simulink model "fec_ber_hw"  (R2020b)
settings: Solver=FixedStepDiscrete  StartTime=0.0  StopTime=T/2  RelTol=1e-3
values from neighbouring files (symbols this model uses):
  aximm_awgn_reset = 0    [setup.m]
  aximm_bit_count_reset = 0    [setup.m]
  aximm_bits = n_blocks * k    (= 3200)    [setup.m]
  aximm_ctrl_word_dec = 0    [setup.m]
  aximm_ctrl_word_enc = 0    [setup.m]
  aximm_enable = 1    [setup.m]
  aximm_length = k * n_blocks    (= 3200)    [setup.m]
  aximm_length_dec = n    (= 160)    [setup.m]
  aximm_length_enc = k    (= 80)    [setup.m]
  aximm_llr_mag_reset = 0    [setup.m]
  aximm_llr_scale = (1/noise_var) * llr_scale    (= 1000)    [setup.m]
  aximm_load_dec = 1    [setup.m]
  aximm_load_enc = 1    [setup.m]
  aximm_noise_std = sqrt(noise_var)    [setup.m]
  aximm_reset = 0    [setup.m]
  d = sqrt(-2*log([0:1/4095:1]))    [setup.m]
  fs = 160e6    (= 160000000)    [setup.m]
  llr_scale = 7.75/7.75    (= 1)    [setup.m]
libraries: simulink x450, hdlsllib x190, commseqgen3 x20, dspsigops x17, lib_rfsoc_fec x5, commblkcod2 x3
(part 20 of 22)

== system fec_ber_hw/Soft Demodulation/SSR Soft Demodulation Lane 1/Soft Demodulation 10/Subsystem2/get_min2 ==
  a : Inport
  b : Inport  Port=2
  Compare To Zero : simulink/Logic and Bit Operations/Compare To Zero  relop=<=  OutDataTypeStr=boolean
  Multiport Switch2 : MultiPortSwitch  DataPortOrder=Zero-based contiguous  Inputs=2  zeroidx=on
  Subtract18 : Sum  Inputs=+-  OutDataTypeStr=fixdt(1,(w+1)*2+2,f*2)  SaturateOnIntegerOverflow=on
  min : Outport
  wires:
  Compare To Zero/1 -> Multiport Switch2/1
  Multiport Switch2/1 -> min/1
  a/1 -> Subtract18/1, Multiport Switch2/3
  b/1 -> Multiport Switch2/2, Subtract18/2
  Subtract18/1 -> Compare To Zero/1

== system fec_ber_hw/Soft Demodulation/SSR Soft Demodulation Lane 1/Soft Demodulation 10/Subsystem2/get_min3 ==
  a : Inport
  b : Inport  Port=2
  Compare To Zero : simulink/Logic and Bit Operations/Compare To Zero  relop=<=  OutDataTypeStr=boolean
  Multiport Switch2 : MultiPortSwitch  DataPortOrder=Zero-based contiguous  Inputs=2  zeroidx=on
  Subtract18 : Sum  Inputs=+-  OutDataTypeStr=fixdt(1,(w+1)*2+2,f*2)  SaturateOnIntegerOverflow=on
  min : Outport
  wires:
  Subtract18/1 -> Compare To Zero/1
  b/1 -> Subtract18/2, Multiport Switch2/2
  a/1 -> Multiport Switch2/3, Subtract18/1
  Multiport Switch2/1 -> min/1
  Compare To Zero/1 -> Multiport Switch2/1

== system fec_ber_hw/Soft Demodulation/SSR Soft Demodulation Lane 1/Soft Demodulation 10/Subsystem2/get_min4 ==
  a : Inport
  b : Inport  Port=2
  Compare To Zero : simulink/Logic and Bit Operations/Compare To Zero  relop=<=  OutDataTypeStr=boolean
  Multiport Switch2 : MultiPortSwitch  DataPortOrder=Zero-based contiguous  Inputs=2  zeroidx=on
  Subtract18 : Sum  Inputs=+-  OutDataTypeStr=fixdt(1,(w+1)*2+2,f*2)  SaturateOnIntegerOverflow=on
  min : Outport
  wires:
  Compare To Zero/1 -> Multiport Switch2/1
  Multiport Switch2/1 -> min/1
  a/1 -> Subtract18/1, Multiport Switch2/3
  b/1 -> Multiport Switch2/2, Subtract18/2
  Subtract18/1 -> Compare To Zero/1

== system fec_ber_hw/Soft Demodulation/SSR Soft Demodulation Lane 1/Soft Demodulation 10/Subsystem2/get_min5 ==
  a : Inport
  b : Inport  Port=2
  Compare To Zero : simulink/Logic and Bit Operations/Compare To Zero  relop=<=  OutDataTypeStr=boolean
  Multiport Switch2 : MultiPortSwitch  DataPortOrder=Zero-based contiguous  Inputs=2  zeroidx=on
  Subtract18 : Sum  Inputs=+-  OutDataTypeStr=fixdt(1,(w+1)*2+2,f*2)  SaturateOnIntegerOverflow=on
  min : Outport
  wires:
  Subtract18/1 -> Compare To Zero/1
  b/1 -> Subtract18/2, Multiport Switch2/2
  a/1 -> Multiport Switch2/3, Subtract18/1
  Multiport Switch2/1 -> min/1
  Compare To Zero/1 -> Multiport Switch2/1

== system fec_ber_hw/Soft Demodulation/SSR Soft Demodulation Lane 1/Soft Demodulation 10/Subsystem2/get_min6 ==
  a : Inport
  b : Inport  Port=2
  Compare To Zero : simulink/Logic and Bit Operations/Compare To Zero  relop=<=  OutDataTypeStr=boolean
  Multiport Switch2 : MultiPortSwitch  DataPortOrder=Zero-based contiguous  Inputs=2  zeroidx=on
  Subtract18 : Sum  Inputs=+-  OutDataTypeStr=fixdt(1,(w+1)*2+2,f*2)  SaturateOnIntegerOverflow=on
  min : Outport
  wires:
  Compare To Zero/1 -> Multiport Switch2/1
  Multiport Switch2/1 -> min/1
  a/1 -> Subtract18/1, Multiport Switch2/3
  b/1 -> Multiport Switch2/2, Subtract18/2
  Subtract18/1 -> Compare To Zero/1

== system fec_ber_hw/Soft Demodulation/SSR Soft Demodulation Lane 1/Soft Demodulation 10/Subsystem2/get_min7 ==
  a : Inport
  b : Inport  Port=2
  Compare To Zero : simulink/Logic and Bit Operations/Compare To Zero  relop=<=  OutDataTypeStr=boolean
  Multiport Switch2 : MultiPortSwitch  DataPortOrder=Zero-based contiguous  Inputs=2  zeroidx=on
  Subtract18 : Sum  Inputs=+-  OutDataTypeStr=fixdt(1,(w+1)*2+2,f*2)  SaturateOnIntegerOverflow=on
  min : Outport
  wires:
  Compare To Zero/1 -> Multiport Switch2/1
  Multiport Switch2/1 -> min/1
  a/1 -> Subtract18/1, Multiport Switch2/3
  b/1 -> Multiport Switch2/2, Subtract18/2
  Subtract18/1 -> Compare To Zero/1

== system fec_ber_hw/Soft Demodulation/SSR Soft Demodulation Lane 1/Soft Demodulation 11/Subsystem1/get_min1 ==
  a : Inport
  b : Inport  Port=2
  Compare To Zero : simulink/Logic and Bit Operations/Compare To Zero  relop=<=  OutDataTypeStr=boolean
  Multiport Switch2 : MultiPortSwitch  DataPortOrder=Zero-based contiguous  Inputs=2  zeroidx=on
  Subtract18 : Sum  Inputs=+-  OutDataTypeStr=fixdt(1,(w+1)*2+2,f*2)  SaturateOnIntegerOverflow=on
  min : Outport
  wires:
  Subtract18/1 -> Compare To Zero/1
  b/1 -> Subtract18/2, Multiport Switch2/2
  a/1 -> Multiport Switch2/3, Subtract18/1
  Multiport Switch2/1 -> min/1
  Compare To Zero/1 -> Multiport Switch2/1

== system fec_ber_hw/Soft Demodulation/SSR Soft Demodulation Lane 1/Soft Demodulation 11/Subsystem1/get_min2 ==
  a : Inport
  b : Inport  Port=2
  Compare To Zero : simulink/Logic and Bit Operations/Compare To Zero  relop=<=  OutDataTypeStr=boolean
  Multiport Switch2 : MultiPortSwitch  DataPortOrder=Zero-based contiguous  Inputs=2  zeroidx=on
  Subtract18 : Sum  Inputs=+-  OutDataTypeStr=fixdt(1,(w+1)*2+2,f*2)  SaturateOnIntegerOverflow=on
  min : Outport
  wires:
  Compare To Zero/1 -> Multiport Switch2/1
  Multiport Switch2/1 -> min/1
  a/1 -> Subtract18/1, Multiport Switch2/3
  b/1 -> Multiport Switch2/2, Subtract18/2
  Subtract18/1 -> Compare To Zero/1

== system fec_ber_hw/Soft Demodulation/SSR Soft Demodulation Lane 1/Soft Demodulation 11/Subsystem1/get_min3 ==
  a : Inport
  b : Inport  Port=2
  Compare To Zero : simulink/Logic and Bit Operations/Compare To Zero  relop=<=  OutDataTypeStr=boolean
  Multiport Switch2 : MultiPortSwitch  DataPortOrder=Zero-based contiguous  Inputs=2  zeroidx=on
  Subtract18 : Sum  Inputs=+-  OutDataTypeStr=fixdt(1,(w+1)*2+2,f*2)  SaturateOnIntegerOverflow=on
  min : Outport
  wires:
  Subtract18/1 -> Compare To Zero/1
  b/1 -> Subtract18/2, Multiport Switch2/2
  a/1 -> Multiport Switch2/3, Subtract18/1
  Multiport Switch2/1 -> min/1
  Compare To Zero/1 -> Multiport Switch2/1

== system fec_ber_hw/Soft Demodulation/SSR Soft Demodulation Lane 1/Soft Demodulation 11/Subsystem1/get_min4 ==
  a : Inport
  b : Inport  Port=2
  Compare To Zero : simulink/Logic and Bit Operations/Compare To Zero  relop=<=  OutDataTypeStr=boolean
  Multiport Switch2 : MultiPortSwitch  DataPortOrder=Zero-based contiguous  Inputs=2  zeroidx=on
  Subtract18 : Sum  Inputs=+-  OutDataTypeStr=fixdt(1,(w+1)*2+2,f*2)  SaturateOnIntegerOverflow=on
  min : Outport
  wires:
  Compare To Zero/1 -> Multiport Switch2/1
  Multiport Switch2/1 -> min/1
  a/1 -> Subtract18/1, Multiport Switch2/3
  b/1 -> Multiport Switch2/2, Subtract18/2
  Subtract18/1 -> Compare To Zero/1

== system fec_ber_hw/Soft Demodulation/SSR Soft Demodulation Lane 1/Soft Demodulation 11/Subsystem1/get_min5 ==
  a : Inport
  b : Inport  Port=2
  Compare To Zero : simulink/Logic and Bit Operations/Compare To Zero  relop=<=  OutDataTypeStr=boolean
  Multiport Switch2 : MultiPortSwitch  DataPortOrder=Zero-based contiguous  Inputs=2  zeroidx=on
  Subtract18 : Sum  Inputs=+-  OutDataTypeStr=fixdt(1,(w+1)*2+2,f*2)  SaturateOnIntegerOverflow=on
  min : Outport
  wires:
  Subtract18/1 -> Compare To Zero/1
  b/1 -> Subtract18/2, Multiport Switch2/2
  a/1 -> Multiport Switch2/3, Subtract18/1
  Multiport Switch2/1 -> min/1
  Compare To Zero/1 -> Multiport Switch2/1

== system fec_ber_hw/Soft Demodulation/SSR Soft Demodulation Lane 1/Soft Demodulation 11/Subsystem1/get_min6 ==
  a : Inport
  b : Inport  Port=2
  Compare To Zero : simulink/Logic and Bit Operations/Compare To Zero  relop=<=  OutDataTypeStr=boolean
  Multiport Switch2 : MultiPortSwitch  DataPortOrder=Zero-based contiguous  Inputs=2  zeroidx=on
  Subtract18 : Sum  Inputs=+-  OutDataTypeStr=fixdt(1,(w+1)*2+2,f*2)  SaturateOnIntegerOverflow=on
  min : Outport
  wires:
  Compare To Zero/1 -> Multiport Switch2/1
  Multiport Switch2/1 -> min/1
  a/1 -> Subtract18/1, Multiport Switch2/3
  b/1 -> Multiport Switch2/2, Subtract18/2
  Subtract18/1 -> Compare To Zero/1

== system fec_ber_hw/Soft Demodulation/SSR Soft Demodulation Lane 1/Soft Demodulation 11/Subsystem1/get_min7 ==
  a : Inport
  b : Inport  Port=2
  Compare To Zero : simulink/Logic and Bit Operations/Compare To Zero  relop=<=  OutDataTypeStr=boolean
  Multiport Switch2 : MultiPortSwitch  DataPortOrder=Zero-based contiguous  Inputs=2  zeroidx=on
  Subtract18 : Sum  Inputs=+-  OutDataTypeStr=fixdt(1,(w+1)*2+2,f*2)  SaturateOnIntegerOverflow=on
  min : Outport
  wires:
  Compare To Zero/1 -> Multiport Switch2/1
  Multiport Switch2/1 -> min/1
  a/1 -> Subtract18/1, Multiport Switch2/3
  b/1 -> Multiport Switch2/2, Subtract18/2
  Subtract18/1 -> Compare To Zero/1

== system fec_ber_hw/Soft Demodulation/SSR Soft Demodulation Lane 1/Soft Demodulation 11/Subsystem2/get_min1 ==
  a : Inport
  b : Inport  Port=2
  Compare To Zero : simulink/Logic and Bit Operations/Compare To Zero  relop=<=  OutDataTypeStr=boolean
  Multiport Switch2 : MultiPortSwitch  DataPortOrder=Zero-based contiguous  Inputs=2  zeroidx=on
  Subtract18 : Sum  Inputs=+-  OutDataTypeStr=fixdt(1,(w+1)*2+2,f*2)  SaturateOnIntegerOverflow=on
  min : Outport
  wires:
  Subtract18/1 -> Compare To Zero/1
  b/1 -> Subtract18/2, Multiport Switch2/2
  a/1 -> Multiport Switch2/3, Subtract18/1
  Multiport Switch2/1 -> min/1
  Compare To Zero/1 -> Multiport Switch2/1

== system fec_ber_hw/Soft Demodulation/SSR Soft Demodulation Lane 1/Soft Demodulation 11/Subsystem2/get_min2 ==
  a : Inport
  b : Inport  Port=2
  Compare To Zero : simulink/Logic and Bit Operations/Compare To Zero  relop=<=  OutDataTypeStr=boolean
  Multiport Switch2 : MultiPortSwitch  DataPortOrder=Zero-based contiguous  Inputs=2  zeroidx=on
  Subtract18 : Sum  Inputs=+-  OutDataTypeStr=fixdt(1,(w+1)*2+2,f*2)  SaturateOnIntegerOverflow=on
  min : Outport
  wires:
  Compare To Zero/1 -> Multiport Switch2/1
  Multiport Switch2/1 -> min/1
  a/1 -> Subtract18/1, Multiport Switch2/3
  b/1 -> Multiport Switch2/2, Subtract18/2
  Subtract18/1 -> Compare To Zero/1

== system fec_ber_hw/Soft Demodulation/SSR Soft Demodulation Lane 1/Soft Demodulation 11/Subsystem2/get_min3 ==
  a : Inport
  b : Inport  Port=2
  Compare To Zero : simulink/Logic and Bit Operations/Compare To Zero  relop=<=  OutDataTypeStr=boolean
  Multiport Switch2 : MultiPortSwitch  DataPortOrder=Zero-based contiguous  Inputs=2  zeroidx=on
  Subtract18 : Sum  Inputs=+-  OutDataTypeStr=fixdt(1,(w+1)*2+2,f*2)  SaturateOnIntegerOverflow=on
  min : Outport
  wires:
  Subtract18/1 -> Compare To Zero/1
  b/1 -> Subtract18/2, Multiport Switch2/2
  a/1 -> Multiport Switch2/3, Subtract18/1
  Multiport Switch2/1 -> min/1
  Compare To Zero/1 -> Multiport Switch2/1

== system fec_ber_hw/Soft Demodulation/SSR Soft Demodulation Lane 1/Soft Demodulation 11/Subsystem2/get_min4 ==
  a : Inport
  b : Inport  Port=2
  Compare To Zero : simulink/Logic and Bit Operations/Compare To Zero  relop=<=  OutDataTypeStr=boolean
  Multiport Switch2 : MultiPortSwitch  DataPortOrder=Zero-based contiguous  Inputs=2  zeroidx=on
  Subtract18 : Sum  Inputs=+-  OutDataTypeStr=fixdt(1,(w+1)*2+2,f*2)  SaturateOnIntegerOverflow=on
  min : Outport
  wires:
  Compare To Zero/1 -> Multiport Switch2/1
  Multiport Switch2/1 -> min/1
  a/1 -> Subtract18/1, Multiport Switch2/3
  b/1 -> Multiport Switch2/2, Subtract18/2
  Subtract18/1 -> Compare To Zero/1

== system fec_ber_hw/Soft Demodulation/SSR Soft Demodulation Lane 1/Soft Demodulation 11/Subsystem2/get_min5 ==
  a : Inport
  b : Inport  Port=2
  Compare To Zero : simulink/Logic and Bit Operations/Compare To Zero  relop=<=  OutDataTypeStr=boolean
  Multiport Switch2 : MultiPortSwitch  DataPortOrder=Zero-based contiguous  Inputs=2  zeroidx=on
  Subtract18 : Sum  Inputs=+-  OutDataTypeStr=fixdt(1,(w+1)*2+2,f*2)  SaturateOnIntegerOverflow=on
  min : Outport
  wires:
  Subtract18/1 -> Compare To Zero/1
  b/1 -> Subtract18/2, Multiport Switch2/2
  a/1 -> Multiport Switch2/3, Subtract18/1
  Multiport Switch2/1 -> min/1
  Compare To Zero/1 -> Multiport Switch2/1

== system fec_ber_hw/Soft Demodulation/SSR Soft Demodulation Lane 1/Soft Demodulation 11/Subsystem2/get_min6 ==
  a : Inport
  b : Inport  Port=2
  Compare To Zero : simulink/Logic and Bit Operations/Compare To Zero  relop=<=  OutDataTypeStr=boolean
  Multiport Switch2 : MultiPortSwitch  DataPortOrder=Zero-based contiguous  Inputs=2  zeroidx=on
  Subtract18 : Sum  Inputs=+-  OutDataTypeStr=fixdt(1,(w+1)*2+2,f*2)  SaturateOnIntegerOverflow=on
  min : Outport
  wires:
  Compare To Zero/1 -> Multiport Switch2/1
  Multiport Switch2/1 -> min/1
  a/1 -> Subtract18/1, Multiport Switch2/3
  b/1 -> Multiport Switch2/2, Subtract18/2
  Subtract18/1 -> Compare To Zero/1

== system fec_ber_hw/Soft Demodulation/SSR Soft Demodulation Lane 1/Soft Demodulation 11/Subsystem2/get_min7 ==
  a : Inport
  b : Inport  Port=2
  Compare To Zero : simulink/Logic and Bit Operations/Compare To Zero  relop=<=  OutDataTypeStr=boolean
  Multiport Switch2 : MultiPortSwitch  DataPortOrder=Zero-based contiguous  Inputs=2  zeroidx=on
  Subtract18 : Sum  Inputs=+-  OutDataTypeStr=fixdt(1,(w+1)*2+2,f*2)  SaturateOnIntegerOverflow=on
  min : Outport
  wires:
  Compare To Zero/1 -> Multiport Switch2/1
  Multiport Switch2/1 -> min/1
  a/1 -> Subtract18/1, Multiport Switch2/3
  b/1 -> Multiport Switch2/2, Subtract18/2
  Subtract18/1 -> Compare To Zero/1

== system fec_ber_hw/Soft Demodulation/SSR Soft Demodulation Lane 1/Soft Demodulation 12/Subsystem1/get_min1 ==
  a : Inport
  b : Inport  Port=2
  Compare To Zero : simulink/Logic and Bit Operations/Compare To Zero  relop=<=  OutDataTypeStr=boolean
  Multiport Switch2 : MultiPortSwitch  DataPortOrder=Zero-based contiguous  Inputs=2  zeroidx=on
  Subtract18 : Sum  Inputs=+-  OutDataTypeStr=fixdt(1,(w+1)*2+2,f*2)  SaturateOnIntegerOverflow=on
  min : Outport
  wires:
  Subtract18/1 -> Compare To Zero/1
  b/1 -> Subtract18/2, Multiport Switch2/2
  a/1 -> Multiport Switch2/3, Subtract18/1
  Multiport Switch2/1 -> min/1
  Compare To Zero/1 -> Multiport Switch2/1

== system fec_ber_hw/Soft Demodulation/SSR Soft Demodulation Lane 1/Soft Demodulation 12/Subsystem1/get_min2 ==
  a : Inport
  b : Inport  Port=2
  Compare To Zero : simulink/Logic and Bit Operations/Compare To Zero  relop=<=  OutDataTypeStr=boolean
  Multiport Switch2 : MultiPortSwitch  DataPortOrder=Zero-based contiguous  Inputs=2  zeroidx=on
  Subtract18 : Sum  Inputs=+-  OutDataTypeStr=fixdt(1,(w+1)*2+2,f*2)  SaturateOnIntegerOverflow=on
  min : Outport
  wires:
  Compare To Zero/1 -> Multiport Switch2/1
  Multiport Switch2/1 -> min/1
  a/1 -> Subtract18/1, Multiport Switch2/3
  b/1 -> Multiport Switch2/2, Subtract18/2
  Subtract18/1 -> Compare To Zero/1

== system fec_ber_hw/Soft Demodulation/SSR Soft Demodulation Lane 1/Soft Demodulation 12/Subsystem1/get_min3 ==
  a : Inport
  b : Inport  Port=2
  Compare To Zero : simulink/Logic and Bit Operations/Compare To Zero  relop=<=  OutDataTypeStr=boolean
  Multiport Switch2 : MultiPortSwitch  DataPortOrder=Zero-based contiguous  Inputs=2  zeroidx=on
  Subtract18 : Sum  Inputs=+-  OutDataTypeStr=fixdt(1,(w+1)*2+2,f*2)  SaturateOnIntegerOverflow=on
  min : Outport
  wires:
  Subtract18/1 -> Compare To Zero/1
  b/1 -> Subtract18/2, Multiport Switch2/2
  a/1 -> Multiport Switch2/3, Subtract18/1
  Multiport Switch2/1 -> min/1
  Compare To Zero/1 -> Multiport Switch2/1

== system fec_ber_hw/Soft Demodulation/SSR Soft Demodulation Lane 1/Soft Demodulation 12/Subsystem1/get_min4 ==
  a : Inport
  b : Inport  Port=2
  Compare To Zero : simulink/Logic and Bit Operations/Compare To Zero  relop=<=  OutDataTypeStr=boolean
  Multiport Switch2 : MultiPortSwitch  DataPortOrder=Zero-based contiguous  Inputs=2  zeroidx=on
  Subtract18 : Sum  Inputs=+-  OutDataTypeStr=fixdt(1,(w+1)*2+2,f*2)  SaturateOnIntegerOverflow=on
  min : Outport
  wires:
  Compare To Zero/1 -> Multiport Switch2/1
  Multiport Switch2/1 -> min/1
  a/1 -> Subtract18/1, Multiport Switch2/3
  b/1 -> Multiport Switch2/2, Subtract18/2
  Subtract18/1 -> Compare To Zero/1

== system fec_ber_hw/Soft Demodulation/SSR Soft Demodulation Lane 1/Soft Demodulation 12/Subsystem1/get_min5 ==
  a : Inport
  b : Inport  Port=2
  Compare To Zero : simulink/Logic and Bit Operations/Compare To Zero  relop=<=  OutDataTypeStr=boolean
  Multiport Switch2 : MultiPortSwitch  DataPortOrder=Zero-based contiguous  Inputs=2  zeroidx=on
  Subtract18 : Sum  Inputs=+-  OutDataTypeStr=fixdt(1,(w+1)*2+2,f*2)  SaturateOnIntegerOverflow=on
  min : Outport
  wires:
  Subtract18/1 -> Compare To Zero/1
  b/1 -> Subtract18/2, Multiport Switch2/2
  a/1 -> Multiport Switch2/3, Subtract18/1
  Multiport Switch2/1 -> min/1
  Compare To Zero/1 -> Multiport Switch2/1

== system fec_ber_hw/Soft Demodulation/SSR Soft Demodulation Lane 1/Soft Demodulation 12/Subsystem1/get_min6 ==
  a : Inport
  b : Inport  Port=2
  Compare To Zero : simulink/Logic and Bit Operations/Compare To Zero  relop=<=  OutDataTypeStr=boolean
  Multiport Switch2 : MultiPortSwitch  DataPortOrder=Zero-based contiguous  Inputs=2  zeroidx=on
  Subtract18 : Sum  Inputs=+-  OutDataTypeStr=fixdt(1,(w+1)*2+2,f*2)  SaturateOnIntegerOverflow=on
  min : Outport
  wires:
  Compare To Zero/1 -> Multiport Switch2/1
  Multiport Switch2/1 -> min/1
  a/1 -> Subtract18/1, Multiport Switch2/3
  b/1 -> Multiport Switch2/2, Subtract18/2
  Subtract18/1 -> Compare To Zero/1

== system fec_ber_hw/Soft Demodulation/SSR Soft Demodulation Lane 1/Soft Demodulation 12/Subsystem1/get_min7 ==
  a : Inport
  b : Inport  Port=2
  Compare To Zero : simulink/Logic and Bit Operations/Compare To Zero  relop=<=  OutDataTypeStr=boolean
  Multiport Switch2 : MultiPortSwitch  DataPortOrder=Zero-based contiguous  Inputs=2  zeroidx=on
  Subtract18 : Sum  Inputs=+-  OutDataTypeStr=fixdt(1,(w+1)*2+2,f*2)  SaturateOnIntegerOverflow=on
  min : Outport
  wires:
  Compare To Zero/1 -> Multiport Switch2/1
  Multiport Switch2/1 -> min/1
  a/1 -> Subtract18/1, Multiport Switch2/3
  b/1 -> Multiport Switch2/2, Subtract18/2
  Subtract18/1 -> Compare To Zero/1

== system fec_ber_hw/Soft Demodulation/SSR Soft Demodulation Lane 1/Soft Demodulation 12/Subsystem2/get_min1 ==
  a : Inport
  b : Inport  Port=2
  Compare To Zero : simulink/Logic and Bit Operations/Compare To Zero  relop=<=  OutDataTypeStr=boolean
  Multiport Switch2 : MultiPortSwitch  DataPortOrder=Zero-based contiguous  Inputs=2  zeroidx=on
  Subtract18 : Sum  Inputs=+-  OutDataTypeStr=fixdt(1,(w+1)*2+2,f*2)  SaturateOnIntegerOverflow=on
  min : Outport
  wires:
  Subtract18/1 -> Compare To Zero/1
  b/1 -> Subtract18/2, Multiport Switch2/2
  a/1 -> Multiport Switch2/3, Subtract18/1
  Multiport Switch2/1 -> min/1
  Compare To Zero/1 -> Multiport Switch2/1

== system fec_ber_hw/Soft Demodulation/SSR Soft Demodulation Lane 1/Soft Demodulation 12/Subsystem2/get_min2 ==
  a : Inport
  b : Inport  Port=2
  Compare To Zero : simulink/Logic and Bit Operations/Compare To Zero  relop=<=  OutDataTypeStr=boolean
  Multiport Switch2 : MultiPortSwitch  DataPortOrder=Zero-based contiguous  Inputs=2  zeroidx=on
  Subtract18 : Sum  Inputs=+-  OutDataTypeStr=fixdt(1,(w+1)*2+2,f*2)  SaturateOnIntegerOverflow=on
  min : Outport
  wires:
  Compare To Zero/1 -> Multiport Switch2/1
  Multiport Switch2/1 -> min/1
  a/1 -> Subtract18/1, Multiport Switch2/3
  b/1 -> Multiport Switch2/2, Subtract18/2
  Subtract18/1 -> Compare To Zero/1

== system fec_ber_hw/Soft Demodulation/SSR Soft Demodulation Lane 1/Soft Demodulation 12/Subsystem2/get_min3 ==
  a : Inport
  b : Inport  Port=2
  Compare To Zero : simulink/Logic and Bit Operations/Compare To Zero  relop=<=  OutDataTypeStr=boolean
  Multiport Switch2 : MultiPortSwitch  DataPortOrder=Zero-based contiguous  Inputs=2  zeroidx=on
  Subtract18 : Sum  Inputs=+-  OutDataTypeStr=fixdt(1,(w+1)*2+2,f*2)  SaturateOnIntegerOverflow=on
  min : Outport
  wires:
  Subtract18/1 -> Compare To Zero/1
  b/1 -> Subtract18/2, Multiport Switch2/2
  a/1 -> Multiport Switch2/3, Subtract18/1
  Multiport Switch2/1 -> min/1
  Compare To Zero/1 -> Multiport Switch2/1

== system fec_ber_hw/Soft Demodulation/SSR Soft Demodulation Lane 1/Soft Demodulation 12/Subsystem2/get_min4 ==
  a : Inport
  b : Inport  Port=2
  Compare To Zero : simulink/Logic and Bit Operations/Compare To Zero  relop=<=  OutDataTypeStr=boolean
  Multiport Switch2 : MultiPortSwitch  DataPortOrder=Zero-based contiguous  Inputs=2  zeroidx=on
  Subtract18 : Sum  Inputs=+-  OutDataTypeStr=fixdt(1,(w+1)*2+2,f*2)  SaturateOnIntegerOverflow=on
  min : Outport
  wires:
  Compare To Zero/1 -> Multiport Switch2/1
  Multiport Switch2/1 -> min/1
  a/1 -> Subtract18/1, Multiport Switch2/3
  b/1 -> Multiport Switch2/2, Subtract18/2
  Subtract18/1 -> Compare To Zero/1

== system fec_ber_hw/Soft Demodulation/SSR Soft Demodulation Lane 1/Soft Demodulation 12/Subsystem2/get_min5 ==
  a : Inport
  b : Inport  Port=2
  Compare To Zero : simulink/Logic and Bit Operations/Compare To Zero  relop=<=  OutDataTypeStr=boolean
  Multiport Switch2 : MultiPortSwitch  DataPortOrder=Zero-based contiguous  Inputs=2  zeroidx=on
  Subtract18 : Sum  Inputs=+-  OutDataTypeStr=fixdt(1,(w+1)*2+2,f*2)  SaturateOnIntegerOverflow=on
  min : Outport
  wires:
  Subtract18/1 -> Compare To Zero/1
  b/1 -> Subtract18/2, Multiport Switch2/2
  a/1 -> Multiport Switch2/3, Subtract18/1
  Multiport Switch2/1 -> min/1
  Compare To Zero/1 -> Multiport Switch2/1

== system fec_ber_hw/Soft Demodulation/SSR Soft Demodulation Lane 1/Soft Demodulation 12/Subsystem2/get_min6 ==
  a : Inport
  b : Inport  Port=2
  Compare To Zero : simulink/Logic and Bit Operations/Compare To Zero  relop=<=  OutDataTypeStr=boolean
  Multiport Switch2 : MultiPortSwitch  DataPortOrder=Zero-based contiguous  Inputs=2  zeroidx=on
  Subtract18 : Sum  Inputs=+-  OutDataTypeStr=fixdt(1,(w+1)*2+2,f*2)  SaturateOnIntegerOverflow=on
  min : Outport
  wires:
  Compare To Zero/1 -> Multiport Switch2/1
  Multiport Switch2/1 -> min/1
  a/1 -> Subtract18/1, Multiport Switch2/3
  b/1 -> Multiport Switch2/2, Subtract18/2
  Subtract18/1 -> Compare To Zero/1

== system fec_ber_hw/Soft Demodulation/SSR Soft Demodulation Lane 1/Soft Demodulation 12/Subsystem2/get_min7 ==
  a : Inport
  b : Inport  Port=2
  Compare To Zero : simulink/Logic and Bit Operations/Compare To Zero  relop=<=  OutDataTypeStr=boolean
  Multiport Switch2 : MultiPortSwitch  DataPortOrder=Zero-based contiguous  Inputs=2  zeroidx=on
  Subtract18 : Sum  Inputs=+-  OutDataTypeStr=fixdt(1,(w+1)*2+2,f*2)  SaturateOnIntegerOverflow=on
  min : Outport
  wires:
  Compare To Zero/1 -> Multiport Switch2/1
  Multiport Switch2/1 -> min/1
  a/1 -> Subtract18/1, Multiport Switch2/3
  b/1 -> Multiport Switch2/2, Subtract18/2
  Subtract18/1 -> Compare To Zero/1

== system fec_ber_hw/Soft Demodulation/SSR Soft Demodulation Lane 1/Soft Demodulation 13/Subsystem1/get_min1 ==
  a : Inport
  b : Inport  Port=2
  Compare To Zero : simulink/Logic and Bit Operations/Compare To Zero  relop=<=  OutDataTypeStr=boolean
  Multiport Switch2 : MultiPortSwitch  DataPortOrder=Zero-based contiguous  Inputs=2  zeroidx=on
  Subtract18 : Sum  Inputs=+-  OutDataTypeStr=fixdt(1,(w+1)*2+2,f*2)  SaturateOnIntegerOverflow=on
  min : Outport
  wires:
  Subtract18/1 -> Compare To Zero/1
  b/1 -> Subtract18/2, Multiport Switch2/2
  a/1 -> Multiport Switch2/3, Subtract18/1
  Multiport Switch2/1 -> min/1
  Compare To Zero/1 -> Multiport Switch2/1

== system fec_ber_hw/Soft Demodulation/SSR Soft Demodulation Lane 1/Soft Demodulation 13/Subsystem1/get_min2 ==
  a : Inport
  b : Inport  Port=2
  Compare To Zero : simulink/Logic and Bit Operations/Compare To Zero  relop=<=  OutDataTypeStr=boolean
  Multiport Switch2 : MultiPortSwitch  DataPortOrder=Zero-based contiguous  Inputs=2  zeroidx=on
  Subtract18 : Sum  Inputs=+-  OutDataTypeStr=fixdt(1,(w+1)*2+2,f*2)  SaturateOnIntegerOverflow=on
  min : Outport
  wires:
  Compare To Zero/1 -> Multiport Switch2/1
  Multiport Switch2/1 -> min/1
  a/1 -> Subtract18/1, Multiport Switch2/3
  b/1 -> Multiport Switch2/2, Subtract18/2
  Subtract18/1 -> Compare To Zero/1

== system fec_ber_hw/Soft Demodulation/SSR Soft Demodulation Lane 1/Soft Demodulation 13/Subsystem1/get_min3 ==
  a : Inport
  b : Inport  Port=2
  Compare To Zero : simulink/Logic and Bit Operations/Compare To Zero  relop=<=  OutDataTypeStr=boolean
  Multiport Switch2 : MultiPortSwitch  DataPortOrder=Zero-based contiguous  Inputs=2  zeroidx=on
  Subtract18 : Sum  Inputs=+-  OutDataTypeStr=fixdt(1,(w+1)*2+2,f*2)  SaturateOnIntegerOverflow=on
  min : Outport
  wires:
  Subtract18/1 -> Compare To Zero/1
  b/1 -> Subtract18/2, Multiport Switch2/2
  a/1 -> Multiport Switch2/3, Subtract18/1
  Multiport Switch2/1 -> min/1
  Compare To Zero/1 -> Multiport Switch2/1

== system fec_ber_hw/Soft Demodulation/SSR Soft Demodulation Lane 1/Soft Demodulation 13/Subsystem1/get_min4 ==
  a : Inport
  b : Inport  Port=2
  Compare To Zero : simulink/Logic and Bit Operations/Compare To Zero  relop=<=  OutDataTypeStr=boolean
  Multiport Switch2 : MultiPortSwitch  DataPortOrder=Zero-based contiguous  Inputs=2  zeroidx=on
  Subtract18 : Sum  Inputs=+-  OutDataTypeStr=fixdt(1,(w+1)*2+2,f*2)  SaturateOnIntegerOverflow=on
  min : Outport
  wires:
  Compare To Zero/1 -> Multiport Switch2/1
  Multiport Switch2/1 -> min/1
  a/1 -> Subtract18/1, Multiport Switch2/3
  b/1 -> Multiport Switch2/2, Subtract18/2
  Subtract18/1 -> Compare To Zero/1

== system fec_ber_hw/Soft Demodulation/SSR Soft Demodulation Lane 1/Soft Demodulation 13/Subsystem1/get_min5 ==
  a : Inport
  b : Inport  Port=2
  Compare To Zero : simulink/Logic and Bit Operations/Compare To Zero  relop=<=  OutDataTypeStr=boolean
  Multiport Switch2 : MultiPortSwitch  DataPortOrder=Zero-based contiguous  Inputs=2  zeroidx=on
  Subtract18 : Sum  Inputs=+-  OutDataTypeStr=fixdt(1,(w+1)*2+2,f*2)  SaturateOnIntegerOverflow=on
  min : Outport
  wires:
  Subtract18/1 -> Compare To Zero/1
  b/1 -> Subtract18/2, Multiport Switch2/2
  a/1 -> Multiport Switch2/3, Subtract18/1
  Multiport Switch2/1 -> min/1
  Compare To Zero/1 -> Multiport Switch2/1

== system fec_ber_hw/Soft Demodulation/SSR Soft Demodulation Lane 1/Soft Demodulation 13/Subsystem1/get_min6 ==
  a : Inport
  b : Inport  Port=2
  Compare To Zero : simulink/Logic and Bit Operations/Compare To Zero  relop=<=  OutDataTypeStr=boolean
  Multiport Switch2 : MultiPortSwitch  DataPortOrder=Zero-based contiguous  Inputs=2  zeroidx=on
  Subtract18 : Sum  Inputs=+-  OutDataTypeStr=fixdt(1,(w+1)*2+2,f*2)  SaturateOnIntegerOverflow=on
  min : Outport
  wires:
  Compare To Zero/1 -> Multiport Switch2/1
  Multiport Switch2/1 -> min/1
  a/1 -> Subtract18/1, Multiport Switch2/3
  b/1 -> Multiport Switch2/2, Subtract18/2
  Subtract18/1 -> Compare To Zero/1

== system fec_ber_hw/Soft Demodulation/SSR Soft Demodulation Lane 1/Soft Demodulation 13/Subsystem1/get_min7 ==
  a : Inport
  b : Inport  Port=2
  Compare To Zero : simulink/Logic and Bit Operations/Compare To Zero  relop=<=  OutDataTypeStr=boolean
  Multiport Switch2 : MultiPortSwitch  DataPortOrder=Zero-based contiguous  Inputs=2  zeroidx=on
  Subtract18 : Sum  Inputs=+-  OutDataTypeStr=fixdt(1,(w+1)*2+2,f*2)  SaturateOnIntegerOverflow=on
  min : Outport
  wires:
  Compare To Zero/1 -> Multiport Switch2/1
  Multiport Switch2/1 -> min/1
  a/1 -> Subtract18/1, Multiport Switch2/3
  b/1 -> Multiport Switch2/2, Subtract18/2
  Subtract18/1 -> Compare To Zero/1

== system fec_ber_hw/Soft Demodulation/SSR Soft Demodulation Lane 1/Soft Demodulation 13/Subsystem2/get_min1 ==
  a : Inport
  b : Inport  Port=2
  Compare To Zero : simulink/Logic and Bit Operations/Compare To Zero  relop=<=  OutDataTypeStr=boolean
  Multiport Switch2 : MultiPortSwitch  DataPortOrder=Zero-based contiguous  Inputs=2  zeroidx=on
  Subtract18 : Sum  Inputs=+-  OutDataTypeStr=fixdt(1,(w+1)*2+2,f*2)  SaturateOnIntegerOverflow=on
  min : Outport
  wires:
  Subtract18/1 -> Compare To Zero/1
  b/1 -> Subtract18/2, Multiport Switch2/2
  a/1 -> Multiport Switch2/3, Subtract18/1
  Multiport Switch2/1 -> min/1
  Compare To Zero/1 -> Multiport Switch2/1

== system fec_ber_hw/Soft Demodulation/SSR Soft Demodulation Lane 1/Soft Demodulation 13/Subsystem2/get_min2 ==
  a : Inport
  b : Inport  Port=2
  Compare To Zero : simulink/Logic and Bit Operations/Compare To Zero  relop=<=  OutDataTypeStr=boolean
  Multiport Switch2 : MultiPortSwitch  DataPortOrder=Zero-based contiguous  Inputs=2  zeroidx=on
  Subtract18 : Sum  Inputs=+-  OutDataTypeStr=fixdt(1,(w+1)*2+2,f*2)  SaturateOnIntegerOverflow=on
  min : Outport
  wires:
  Compare To Zero/1 -> Multiport Switch2/1
  Multiport Switch2/1 -> min/1
  a/1 -> Subtract18/1, Multiport Switch2/3
  b/1 -> Multiport Switch2/2, Subtract18/2
  Subtract18/1 -> Compare To Zero/1

== system fec_ber_hw/Soft Demodulation/SSR Soft Demodulation Lane 1/Soft Demodulation 13/Subsystem2/get_min3 ==
  a : Inport
  b : Inport  Port=2
  Compare To Zero : simulink/Logic and Bit Operations/Compare To Zero  relop=<=  OutDataTypeStr=boolean
  Multiport Switch2 : MultiPortSwitch  DataPortOrder=Zero-based contiguous  Inputs=2  zeroidx=on
  Subtract18 : Sum  Inputs=+-  OutDataTypeStr=fixdt(1,(w+1)*2+2,f*2)  SaturateOnIntegerOverflow=on
  min : Outport
  wires:
  Subtract18/1 -> Compare To Zero/1
  b/1 -> Subtract18/2, Multiport Switch2/2
  a/1 -> Multiport Switch2/3, Subtract18/1
  Multiport Switch2/1 -> min/1
  Compare To Zero/1 -> Multiport Switch2/1

== system fec_ber_hw/Soft Demodulation/SSR Soft Demodulation Lane 1/Soft Demodulation 13/Subsystem2/get_min4 ==
  a : Inport
  b : Inport  Port=2
  Compare To Zero : simulink/Logic and Bit Operations/Compare To Zero  relop=<=  OutDataTypeStr=boolean
  Multiport Switch2 : MultiPortSwitch  DataPortOrder=Zero-based contiguous  Inputs=2  zeroidx=on
  Subtract18 : Sum  Inputs=+-  OutDataTypeStr=fixdt(1,(w+1)*2+2,f*2)  SaturateOnIntegerOverflow=on
  min : Outport
  wires:
  Compare To Zero/1 -> Multiport Switch2/1
  Multiport Switch2/1 -> min/1
  a/1 -> Subtract18/1, Multiport Switch2/3
  b/1 -> Multiport Switch2/2, Subtract18/2
  Subtract18/1 -> Compare To Zero/1

== system fec_ber_hw/Soft Demodulation/SSR Soft Demodulation Lane 1/Soft Demodulation 13/Subsystem2/get_min5 ==
  a : Inport
  b : Inport  Port=2
  Compare To Zero : simulink/Logic and Bit Operations/Compare To Zero  relop=<=  OutDataTypeStr=boolean
  Multiport Switch2 : MultiPortSwitch  DataPortOrder=Zero-based contiguous  Inputs=2  zeroidx=on
  Subtract18 : Sum  Inputs=+-  OutDataTypeStr=fixdt(1,(w+1)*2+2,f*2)  SaturateOnIntegerOverflow=on
  min : Outport
  wires:
  Subtract18/1 -> Compare To Zero/1
  b/1 -> Subtract18/2, Multiport Switch2/2
  a/1 -> Multiport Switch2/3, Subtract18/1
  Multiport Switch2/1 -> min/1
  Compare To Zero/1 -> Multiport Switch2/1

== system fec_ber_hw/Soft Demodulation/SSR Soft Demodulation Lane 1/Soft Demodulation 13/Subsystem2/get_min6 ==
  a : Inport
  b : Inport  Port=2
  Compare To Zero : simulink/Logic and Bit Operations/Compare To Zero  relop=<=  OutDataTypeStr=boolean
  Multiport Switch2 : MultiPortSwitch  DataPortOrder=Zero-based contiguous  Inputs=2  zeroidx=on
  Subtract18 : Sum  Inputs=+-  OutDataTypeStr=fixdt(1,(w+1)*2+2,f*2)  SaturateOnIntegerOverflow=on
  min : Outport
  wires:
  Compare To Zero/1 -> Multiport Switch2/1
  Multiport Switch2/1 -> min/1
  a/1 -> Subtract18/1, Multiport Switch2/3
  b/1 -> Multiport Switch2/2, Subtract18/2
  Subtract18/1 -> Compare To Zero/1

== system fec_ber_hw/Soft Demodulation/SSR Soft Demodulation Lane 1/Soft Demodulation 13/Subsystem2/get_min7 ==
  a : Inport
  b : Inport  Port=2
  Compare To Zero : simulink/Logic and Bit Operations/Compare To Zero  relop=<=  OutDataTypeStr=boolean
  Multiport Switch2 : MultiPortSwitch  DataPortOrder=Zero-based contiguous  Inputs=2  zeroidx=on
  Subtract18 : Sum  Inputs=+-  OutDataTypeStr=fixdt(1,(w+1)*2+2,f*2)  SaturateOnIntegerOverflow=on
  min : Outport
  wires:
  Compare To Zero/1 -> Multiport Switch2/1
  Multiport Switch2/1 -> min/1
  a/1 -> Subtract18/1, Multiport Switch2/3
  b/1 -> Multiport Switch2/2, Subtract18/2
  Subtract18/1 -> Compare To Zero/1

== system fec_ber_hw/Soft Demodulation/SSR Soft Demodulation Lane 1/Soft Demodulation 14/Subsystem1/get_min1 ==
  a : Inport
  b : Inport  Port=2
  Compare To Zero : simulink/Logic and Bit Operations/Compare To Zero  relop=<=  OutDataTypeStr=boolean
  Multiport Switch2 : MultiPortSwitch  DataPortOrder=Zero-based contiguous  Inputs=2  zeroidx=on
  Subtract18 : Sum  Inputs=+-  OutDataTypeStr=fixdt(1,(w+1)*2+2,f*2)  SaturateOnIntegerOverflow=on
  min : Outport
  wires:
  Subtract18/1 -> Compare To Zero/1
  b/1 -> Subtract18/2, Multiport Switch2/2
  a/1 -> Multiport Switch2/3, Subtract18/1
  Multiport Switch2/1 -> min/1
  Compare To Zero/1 -> Multiport Switch2/1

== system fec_ber_hw/Soft Demodulation/SSR Soft Demodulation Lane 1/Soft Demodulation 14/Subsystem1/get_min2 ==
  a : Inport
  b : Inport  Port=2
  Compare To Zero : simulink/Logic and Bit Operations/Compare To Zero  relop=<=  OutDataTypeStr=boolean
  Multiport Switch2 : MultiPortSwitch  DataPortOrder=Zero-based contiguous  Inputs=2  zeroidx=on
  Subtract18 : Sum  Inputs=+-  OutDataTypeStr=fixdt(1,(w+1)*2+2,f*2)  SaturateOnIntegerOverflow=on
  min : Outport
  wires:
  Compare To Zero/1 -> Multiport Switch2/1
  Multiport Switch2/1 -> min/1
  a/1 -> Subtract18/1, Multiport Switch2/3
  b/1 -> Multiport Switch2/2, Subtract18/2
  Subtract18/1 -> Compare To Zero/1

== system fec_ber_hw/Soft Demodulation/SSR Soft Demodulation Lane 1/Soft Demodulation 14/Subsystem1/get_min3 ==
  a : Inport
  b : Inport  Port=2
  Compare To Zero : simulink/Logic and Bit Operations/Compare To Zero  relop=<=  OutDataTypeStr=boolean
  Multiport Switch2 : MultiPortSwitch  DataPortOrder=Zero-based contiguous  Inputs=2  zeroidx=on
  Subtract18 : Sum  Inputs=+-  OutDataTypeStr=fixdt(1,(w+1)*2+2,f*2)  SaturateOnIntegerOverflow=on
  min : Outport
  wires:
  Subtract18/1 -> Compare To Zero/1
  b/1 -> Subtract18/2, Multiport Switch2/2
  a/1 -> Multiport Switch2/3, Subtract18/1
  Multiport Switch2/1 -> min/1
  Compare To Zero/1 -> Multiport Switch2/1

== system fec_ber_hw/Soft Demodulation/SSR Soft Demodulation Lane 1/Soft Demodulation 14/Subsystem1/get_min4 ==
  a : Inport
  b : Inport  Port=2
  Compare To Zero : simulink/Logic and Bit Operations/Compare To Zero  relop=<=  OutDataTypeStr=boolean
  Multiport Switch2 : MultiPortSwitch  DataPortOrder=Zero-based contiguous  Inputs=2  zeroidx=on
  Subtract18 : Sum  Inputs=+-  OutDataTypeStr=fixdt(1,(w+1)*2+2,f*2)  SaturateOnIntegerOverflow=on
  min : Outport
  wires:
  Compare To Zero/1 -> Multiport Switch2/1
  Multiport Switch2/1 -> min/1
  a/1 -> Subtract18/1, Multiport Switch2/3
  b/1 -> Multiport Switch2/2, Subtract18/2
  Subtract18/1 -> Compare To Zero/1

== system fec_ber_hw/Soft Demodulation/SSR Soft Demodulation Lane 1/Soft Demodulation 14/Subsystem1/get_min5 ==
  a : Inport
  b : Inport  Port=2
  Compare To Zero : simulink/Logic and Bit Operations/Compare To Zero  relop=<=  OutDataTypeStr=boolean
  Multiport Switch2 : MultiPortSwitch  DataPortOrder=Zero-based contiguous  Inputs=2  zeroidx=on
  Subtract18 : Sum  Inputs=+-  OutDataTypeStr=fixdt(1,(w+1)*2+2,f*2)  SaturateOnIntegerOverflow=on
  min : Outport
  wires:
  Subtract18/1 -> Compare To Zero/1
  b/1 -> Subtract18/2, Multiport Switch2/2
  a/1 -> Multiport Switch2/3, Subtract18/1
  Multiport Switch2/1 -> min/1
  Compare To Zero/1 -> Multiport Switch2/1

== system fec_ber_hw/Soft Demodulation/SSR Soft Demodulation Lane 1/Soft Demodulation 14/Subsystem1/get_min6 ==
  a : Inport
  b : Inport  Port=2
  Compare To Zero : simulink/Logic and Bit Operations/Compare To Zero  relop=<=  OutDataTypeStr=boolean
  Multiport Switch2 : MultiPortSwitch  DataPortOrder=Zero-based contiguous  Inputs=2  zeroidx=on
  Subtract18 : Sum  Inputs=+-  OutDataTypeStr=fixdt(1,(w+1)*2+2,f*2)  SaturateOnIntegerOverflow=on
  min : Outport
  wires:
  Compare To Zero/1 -> Multiport Switch2/1
  Multiport Switch2/1 -> min/1
  a/1 -> Subtract18/1, Multiport Switch2/3
  b/1 -> Multiport Switch2/2, Subtract18/2
  Subtract18/1 -> Compare To Zero/1

== system fec_ber_hw/Soft Demodulation/SSR Soft Demodulation Lane 1/Soft Demodulation 14/Subsystem1/get_min7 ==
  a : Inport
  b : Inport  Port=2
  Compare To Zero : simulink/Logic and Bit Operations/Compare To Zero  relop=<=  OutDataTypeStr=boolean
  Multiport Switch2 : MultiPortSwitch  DataPortOrder=Zero-based contiguous  Inputs=2  zeroidx=on
  Subtract18 : Sum  Inputs=+-  OutDataTypeStr=fixdt(1,(w+1)*2+2,f*2)  SaturateOnIntegerOverflow=on
  min : Outport
  wires:
  Compare To Zero/1 -> Multiport Switch2/1
  Multiport Switch2/1 -> min/1
  a/1 -> Subtract18/1, Multiport Switch2/3
  b/1 -> Multiport Switch2/2, Subtract18/2
  Subtract18/1 -> Compare To Zero/1

== system fec_ber_hw/Soft Demodulation/SSR Soft Demodulation Lane 1/Soft Demodulation 14/Subsystem2/get_min1 ==
  a : Inport
  b : Inport  Port=2
  Compare To Zero : simulink/Logic and Bit Operations/Compare To Zero  relop=<=  OutDataTypeStr=boolean
  Multiport Switch2 : MultiPortSwitch  DataPortOrder=Zero-based contiguous  Inputs=2  zeroidx=on
  Subtract18 : Sum  Inputs=+-  OutDataTypeStr=fixdt(1,(w+1)*2+2,f*2)  SaturateOnIntegerOverflow=on
  min : Outport
  wires:
  Subtract18/1 -> Compare To Zero/1
  b/1 -> Subtract18/2, Multiport Switch2/2
  a/1 -> Multiport Switch2/3, Subtract18/1
  Multiport Switch2/1 -> min/1
  Compare To Zero/1 -> Multiport Switch2/1

== system fec_ber_hw/Soft Demodulation/SSR Soft Demodulation Lane 1/Soft Demodulation 14/Subsystem2/get_min2 ==
  a : Inport
  b : Inport  Port=2
  Compare To Zero : simulink/Logic and Bit Operations/Compare To Zero  relop=<=  OutDataTypeStr=boolean
  Multiport Switch2 : MultiPortSwitch  DataPortOrder=Zero-based contiguous  Inputs=2  zeroidx=on
  Subtract18 : Sum  Inputs=+-  OutDataTypeStr=fixdt(1,(w+1)*2+2,f*2)  SaturateOnIntegerOverflow=on
  min : Outport
  wires:
  Compare To Zero/1 -> Multiport Switch2/1
  Multiport Switch2/1 -> min/1
  a/1 -> Subtract18/1, Multiport Switch2/3
  b/1 -> Multiport Switch2/2, Subtract18/2
  Subtract18/1 -> Compare To Zero/1

== system fec_ber_hw/Soft Demodulation/SSR Soft Demodulation Lane 1/Soft Demodulation 14/Subsystem2/get_min3 ==
  a : Inport
  b : Inport  Port=2
  Compare To Zero : simulink/Logic and Bit Operations/Compare To Zero  relop=<=  OutDataTypeStr=boolean
  Multiport Switch2 : MultiPortSwitch  DataPortOrder=Zero-based contiguous  Inputs=2  zeroidx=on
  Subtract18 : Sum  Inputs=+-  OutDataTypeStr=fixdt(1,(w+1)*2+2,f*2)  SaturateOnIntegerOverflow=on
  min : Outport
  wires:
  Subtract18/1 -> Compare To Zero/1
  b/1 -> Subtract18/2, Multiport Switch2/2
  a/1 -> Multiport Switch2/3, Subtract18/1
  Multiport Switch2/1 -> min/1
  Compare To Zero/1 -> Multiport Switch2/1

== system fec_ber_hw/Soft Demodulation/SSR Soft Demodulation Lane 1/Soft Demodulation 14/Subsystem2/get_min4 ==
  a : Inport
  b : Inport  Port=2
  Compare To Zero : simulink/Logic and Bit Operations/Compare To Zero  relop=<=  OutDataTypeStr=boolean
  Multiport Switch2 : MultiPortSwitch  DataPortOrder=Zero-based contiguous  Inputs=2  zeroidx=on
  Subtract18 : Sum  Inputs=+-  OutDataTypeStr=fixdt(1,(w+1)*2+2,f*2)  SaturateOnIntegerOverflow=on
  min : Outport
  wires:
  Compare To Zero/1 -> Multiport Switch2/1
  Multiport Switch2/1 -> min/1
  a/1 -> Subtract18/1, Multiport Switch2/3
  b/1 -> Multiport Switch2/2, Subtract18/2
  Subtract18/1 -> Compare To Zero/1

== system fec_ber_hw/Soft Demodulation/SSR Soft Demodulation Lane 1/Soft Demodulation 14/Subsystem2/get_min5 ==
  a : Inport
  b : Inport  Port=2
  Compare To Zero : simulink/Logic and Bit Operations/Compare To Zero  relop=<=  OutDataTypeStr=boolean
  Multiport Switch2 : MultiPortSwitch  DataPortOrder=Zero-based contiguous  Inputs=2  zeroidx=on
  Subtract18 : Sum  Inputs=+-  OutDataTypeStr=fixdt(1,(w+1)*2+2,f*2)  SaturateOnIntegerOverflow=on
  min : Outport
  wires:
  Subtract18/1 -> Compare To Zero/1
  b/1 -> Subtract18/2, Multiport Switch2/2
  a/1 -> Multiport Switch2/3, Subtract18/1
  Multiport Switch2/1 -> min/1
  Compare To Zero/1 -> Multiport Switch2/1

== system fec_ber_hw/Soft Demodulation/SSR Soft Demodulation Lane 1/Soft Demodulation 14/Subsystem2/get_min6 ==
  a : Inport
  b : Inport  Port=2
  Compare To Zero : simulink/Logic and Bit Operations/Compare To Zero  relop=<=  OutDataTypeStr=boolean
  Multiport Switch2 : MultiPortSwitch  DataPortOrder=Zero-based contiguous  Inputs=2  zeroidx=on
  Subtract18 : Sum  Inputs=+-  OutDataTypeStr=fixdt(1,(w+1)*2+2,f*2)  SaturateOnIntegerOverflow=on
  min : Outport
  wires:
  Compare To Zero/1 -> Multiport Switch2/1
  Multiport Switch2/1 -> min/1
  a/1 -> Subtract18/1, Multiport Switch2/3
  b/1 -> Multiport Switch2/2, Subtract18/2
  Subtract18/1 -> Compare To Zero/1

== system fec_ber_hw/Soft Demodulation/SSR Soft Demodulation Lane 1/Soft Demodulation 14/Subsystem2/get_min7 ==
  a : Inport
  b : Inport  Port=2
  Compare To Zero : simulink/Logic and Bit Operations/Compare To Zero  relop=<=  OutDataTypeStr=boolean
  Multiport Switch2 : MultiPortSwitch  DataPortOrder=Zero-based contiguous  Inputs=2  zeroidx=on
  Subtract18 : Sum  Inputs=+-  OutDataTypeStr=fixdt(1,(w+1)*2+2,f*2)  SaturateOnIntegerOverflow=on
  min : Outport
  wires:
  Compare To Zero/1 -> Multiport Switch2/1
  Multiport Switch2/1 -> min/1
  a/1 -> Subtract18/1, Multiport Switch2/3
  b/1 -> Multiport Switch2/2, Subtract18/2
  Subtract18/1 -> Compare To Zero/1

== system fec_ber_hw/Soft Demodulation/SSR Soft Demodulation Lane 1/Soft Demodulation 15/Subsystem1/get_min1 ==
  a : Inport
  b : Inport  Port=2
  Compare To Zero : simulink/Logic and Bit Operations/Compare To Zero  relop=<=  OutDataTypeStr=boolean
  Multiport Switch2 : MultiPortSwitch  DataPortOrder=Zero-based contiguous  Inputs=2  zeroidx=on
  Subtract18 : Sum  Inputs=+-  OutDataTypeStr=fixdt(1,(w+1)*2+2,f*2)  SaturateOnIntegerOverflow=on
  min : Outport
  wires:
  Subtract18/1 -> Compare To Zero/1
  b/1 -> Subtract18/2, Multiport Switch2/2
  a/1 -> Multiport Switch2/3, Subtract18/1
  Multiport Switch2/1 -> min/1
  Compare To Zero/1 -> Multiport Switch2/1

== system fec_ber_hw/Soft Demodulation/SSR Soft Demodulation Lane 1/Soft Demodulation 15/Subsystem1/get_min2 ==
  a : Inport
  b : Inport  Port=2
  Compare To Zero : simulink/Logic and Bit Operations/Compare To Zero  relop=<=  OutDataTypeStr=boolean
  Multiport Switch2 : MultiPortSwitch  DataPortOrder=Zero-based contiguous  Inputs=2  zeroidx=on
  Subtract18 : Sum  Inputs=+-  OutDataTypeStr=fixdt(1,(w+1)*2+2,f*2)  SaturateOnIntegerOverflow=on
  min : Outport
  wires:
  Compare To Zero/1 -> Multiport Switch2/1
  Multiport Switch2/1 -> min/1
  a/1 -> Subtract18/1, Multiport Switch2/3
  b/1 -> Multiport Switch2/2, Subtract18/2
  Subtract18/1 -> Compare To Zero/1

== system fec_ber_hw/Soft Demodulation/SSR Soft Demodulation Lane 1/Soft Demodulation 15/Subsystem1/get_min3 ==
  a : Inport
  b : Inport  Port=2
  Compare To Zero : simulink/Logic and Bit Operations/Compare To Zero  relop=<=  OutDataTypeStr=boolean
  Multiport Switch2 : MultiPortSwitch  DataPortOrder=Zero-based contiguous  Inputs=2  zeroidx=on
  Subtract18 : Sum  Inputs=+-  OutDataTypeStr=fixdt(1,(w+1)*2+2,f*2)  SaturateOnIntegerOverflow=on
  min : Outport
  wires:
  Subtract18/1 -> Compare To Zero/1
  b/1 -> Subtract18/2, Multiport Switch2/2
  a/1 -> Multiport Switch2/3, Subtract18/1
  Multiport Switch2/1 -> min/1
  Compare To Zero/1 -> Multiport Switch2/1

== system fec_ber_hw/Soft Demodulation/SSR Soft Demodulation Lane 1/Soft Demodulation 15/Subsystem1/get_min4 ==
  a : Inport
  b : Inport  Port=2
  Compare To Zero : simulink/Logic and Bit Operations/Compare To Zero  relop=<=  OutDataTypeStr=boolean
  Multiport Switch2 : MultiPortSwitch  DataPortOrder=Zero-based contiguous  Inputs=2  zeroidx=on
  Subtract18 : Sum  Inputs=+-  OutDataTypeStr=fixdt(1,(w+1)*2+2,f*2)  SaturateOnIntegerOverflow=on
  min : Outport
  wires:
  Compare To Zero/1 -> Multiport Switch2/1
  Multiport Switch2/1 -> min/1
  a/1 -> Subtract18/1, Multiport Switch2/3
  b/1 -> Multiport Switch2/2, Subtract18/2
  Subtract18/1 -> Compare To Zero/1

== system fec_ber_hw/Soft Demodulation/SSR Soft Demodulation Lane 1/Soft Demodulation 15/Subsystem1/get_min5 ==
  a : Inport
  b : Inport  Port=2
  Compare To Zero : simulink/Logic and Bit Operations/Compare To Zero  relop=<=  OutDataTypeStr=boolean
  Multiport Switch2 : MultiPortSwitch  DataPortOrder=Zero-based contiguous  Inputs=2  zeroidx=on
  Subtract18 : Sum  Inputs=+-  OutDataTypeStr=fixdt(1,(w+1)*2+2,f*2)  SaturateOnIntegerOverflow=on
  min : Outport
  wires:
  Subtract18/1 -> Compare To Zero/1
  b/1 -> Subtract18/2, Multiport Switch2/2
  a/1 -> Multiport Switch2/3, Subtract18/1
  Multiport Switch2/1 -> min/1
  Compare To Zero/1 -> Multiport Switch2/1

== system fec_ber_hw/Soft Demodulation/SSR Soft Demodulation Lane 1/Soft Demodulation 15/Subsystem1/get_min6 ==
  a : Inport
  b : Inport  Port=2
  Compare To Zero : simulink/Logic and Bit Operations/Compare To Zero  relop=<=  OutDataTypeStr=boolean
  Multiport Switch2 : MultiPortSwitch  DataPortOrder=Zero-based contiguous  Inputs=2  zeroidx=on
  Subtract18 : Sum  Inputs=+-  OutDataTypeStr=fixdt(1,(w+1)*2+2,f*2)  SaturateOnIntegerOverflow=on
  min : Outport
  wires:
  Compare To Zero/1 -> Multiport Switch2/1
  Multiport Switch2/1 -> min/1
  a/1 -> Subtract18/1, Multiport Switch2/3
  b/1 -> Multiport Switch2/2, Subtract18/2
  Subtract18/1 -> Compare To Zero/1

== system fec_ber_hw/Soft Demodulation/SSR Soft Demodulation Lane 1/Soft Demodulation 15/Subsystem1/get_min7 ==
  a : Inport
  b : Inport  Port=2
  Compare To Zero : simulink/Logic and Bit Operations/Compare To Zero  relop=<=  OutDataTypeStr=boolean
  Multiport Switch2 : MultiPortSwitch  DataPortOrder=Zero-based contiguous  Inputs=2  zeroidx=on
  Subtract18 : Sum  Inputs=+-  OutDataTypeStr=fixdt(1,(w+1)*2+2,f*2)  SaturateOnIntegerOverflow=on
  min : Outport
  wires:
  Compare To Zero/1 -> Multiport Switch2/1
  Multiport Switch2/1 -> min/1
  a/1 -> Subtract18/1, Multiport Switch2/3
  b/1 -> Multiport Switch2/2, Subtract18/2
  Subtract18/1 -> Compare To Zero/1

== system fec_ber_hw/Soft Demodulation/SSR Soft Demodulation Lane 1/Soft Demodulation 15/Subsystem2/get_min1 ==
  a : Inport
  b : Inport  Port=2
  Compare To Zero : simulink/Logic and Bit Operations/Compare To Zero  relop=<=  OutDataTypeStr=boolean
  Multiport Switch2 : MultiPortSwitch  DataPortOrder=Zero-based contiguous  Inputs=2  zeroidx=on
  Subtract18 : Sum  Inputs=+-  OutDataTypeStr=fixdt(1,(w+1)*2+2,f*2)  SaturateOnIntegerOverflow=on
  min : Outport
  wires:
  Subtract18/1 -> Compare To Zero/1
  b/1 -> Subtract18/2, Multiport Switch2/2
  a/1 -> Multiport Switch2/3, Subtract18/1
  Multiport Switch2/1 -> min/1
  Compare To Zero/1 -> Multiport Switch2/1

== system fec_ber_hw/Soft Demodulation/SSR Soft Demodulation Lane 1/Soft Demodulation 15/Subsystem2/get_min2 ==
  a : Inport
  b : Inport  Port=2
  Compare To Zero : simulink/Logic and Bit Operations/Compare To Zero  relop=<=  OutDataTypeStr=boolean
  Multiport Switch2 : MultiPortSwitch  DataPortOrder=Zero-based contiguous  Inputs=2  zeroidx=on
  Subtract18 : Sum  Inputs=+-  OutDataTypeStr=fixdt(1,(w+1)*2+2,f*2)  SaturateOnIntegerOverflow=on
  min : Outport
  wires:
  Compare To Zero/1 -> Multiport Switch2/1
  Multiport Switch2/1 -> min/1
  a/1 -> Subtract18/1, Multiport Switch2/3
  b/1 -> Multiport Switch2/2, Subtract18/2
  Subtract18/1 -> Compare To Zero/1

== system fec_ber_hw/Soft Demodulation/SSR Soft Demodulation Lane 1/Soft Demodulation 15/Subsystem2/get_min3 ==
  a : Inport
  b : Inport  Port=2
  Compare To Zero : simulink/Logic and Bit Operations/Compare To Zero  relop=<=  OutDataTypeStr=boolean
  Multiport Switch2 : MultiPortSwitch  DataPortOrder=Zero-based contiguous  Inputs=2  zeroidx=on
  Subtract18 : Sum  Inputs=+-  OutDataTypeStr=fixdt(1,(w+1)*2+2,f*2)  SaturateOnIntegerOverflow=on
  min : Outport
  wires:
  Subtract18/1 -> Compare To Zero/1
  b/1 -> Subtract18/2, Multiport Switch2/2
  a/1 -> Multiport Switch2/3, Subtract18/1
  Multiport Switch2/1 -> min/1
  Compare To Zero/1 -> Multiport Switch2/1

== system fec_ber_hw/Soft Demodulation/SSR Soft Demodulation Lane 1/Soft Demodulation 15/Subsystem2/get_min4 ==
  a : Inport
  b : Inport  Port=2
  Compare To Zero : simulink/Logic and Bit Operations/Compare To Zero  relop=<=  OutDataTypeStr=boolean
  Multiport Switch2 : MultiPortSwitch  DataPortOrder=Zero-based contiguous  Inputs=2  zeroidx=on
  Subtract18 : Sum  Inputs=+-  OutDataTypeStr=fixdt(1,(w+1)*2+2,f*2)  SaturateOnIntegerOverflow=on
  min : Outport
  wires:
  Compare To Zero/1 -> Multiport Switch2/1
  Multiport Switch2/1 -> min/1
  a/1 -> Subtract18/1, Multiport Switch2/3
  b/1 -> Multiport Switch2/2, Subtract18/2
  Subtract18/1 -> Compare To Zero/1
